simulink model "StepperMotor_time_solver_curve_caratteristiche"  (R2023b)
settings: Solver=FixedStepDiscrete  StartTime=0.0  StopTime=0.25  FixedStep=Ts  MaxStep=2e-6  EnableMultiTasking=on
PreLoadFcn:
  | assignin('base','Ts',1e-6);
InitFcn:
  | Ts=1e-6;
undefined symbols (not defined in the file or in its folder): DiscIntNeverNeededParam
libraries: spsUniversalBridgeLib x2, spsCurrentMeasurementLib x2, spsDCVoltageSourceLib x1, spsStepperMotorLib x1, SignalEditorBlockLib x1, spspowerguiLib x1
settings Model: Creator=The MathWorks, Inc.  LastModifiedBy=simon
settings SolverCC: AlgebraicLoopSolver=TrustRegion
settings DataIOCC: LimitDataPoints=on  SaveFormat=Array  ReturnWorkspaceOutputs=off
settings OptimizationCC: ExpressionDepthLimit=2147483647  InitFltsAndDblsToZero=on  LifeSpan=inf
settings DebuggingCC: UnderspecifiedInitializationDetection=Classic  MergeDetectMultiDrivingBlocksExec=none  SignalResolutionControl=TryResolveAllWithWarning  SolverPrmCheckMsg=warning  FcnCallInpInsideContextMsg=warning  UnconnectedInputMsg=warning  UnconnectedOutputMsg=warning  UnconnectedLineMsg=warning  StateNameClashWarn=warning  SubsystemReferenceDiagnosticForUnitTest=warning  SFUnexpectedBacktrackingDiag=warning  SFNoUnconditionalDefaultTransitionDiag=warning  SFExecutionAtInitializationDiag=none  ArithmeticOperatorsInVariantConditions=warning
settings HardwareCC: ProdBitPerPointer=32  ProdBitPerSizeT=32  ProdBitPerPtrDiffT=32  ProdLargestAtomicFloat=None  ProdIntDivRoundTo=Undefined  ProdEndianess=Unspecified  ProdWordSize=32  ProdHWDeviceType=32-bit Generic
settings ModelReferenceCC: EnableRefExpFcnMdlSchedulingChecks=on  PropagateSignalLabelsOutOfModel=off
settings SFSimCC: SimUseLocalCustomCode=off  CustomCodeUndefinedFunction=UseInterfaceOnly
settings RTWCC: RTWUseLocalCustomCode=off  DLArmComputeVersion=19.05
settings CodeAppCC: StateflowObjectComments=on
settings GRTTargetCC: TargetLangStandard=C89/C90 (ANSI)  CombineOutputUpdateFcns=off  GRTInterface=on
settings ConfigComp: CovMetricSettings=dw  CovSaveCumulativeToWorkspaceVar=on  CovSaveSingleToWorkspaceVar=on  CovExternalEMLEnable=off  CovSFcnEnable=off
settings SimscapeCC: SimscapeNormalizeSystem=off

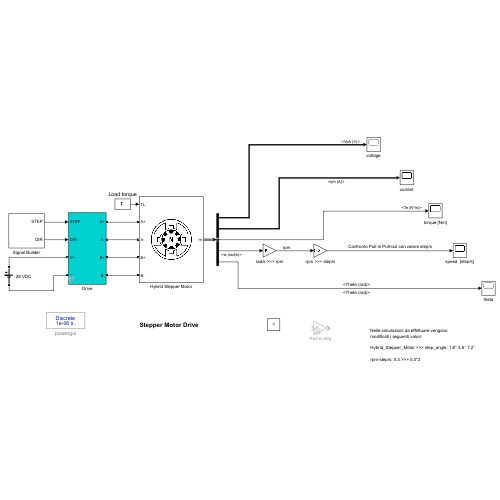
[thumbnail: Simulink's stored preview of the top-level diagram]
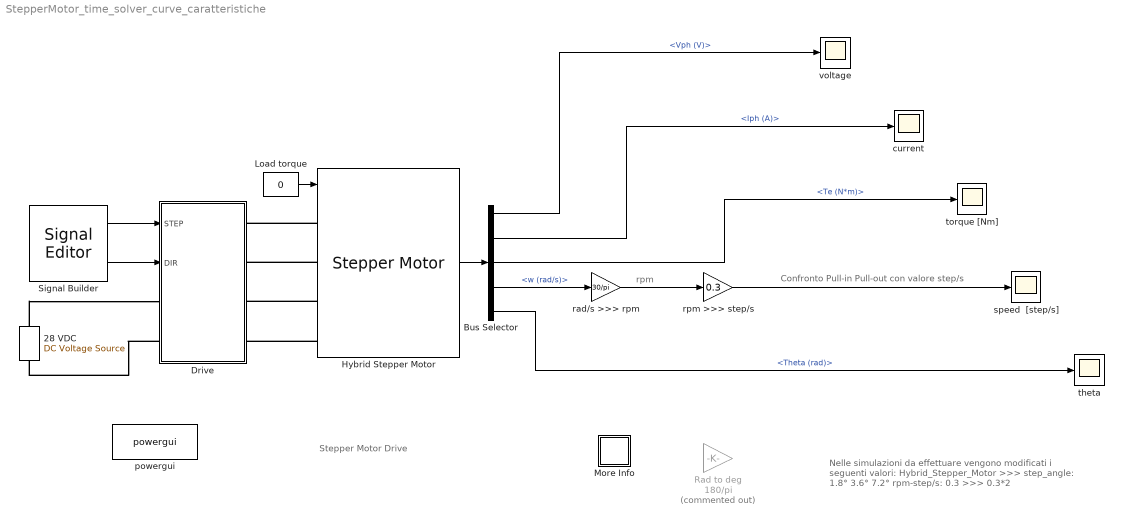
== system StepperMotor_time_solver_curve_caratteristiche ==
  note: Nelle simulazioni da effettuare vengono
      | modificati i seguenti valori:
      |
      | Hybrid_Stepper_Motor >>> step_angle: 1.8° 3.6° 7.2°
      |
      | rpm-step/s: 0.3 >>> 0.3*2
  note: Confronto Pull-in Pull-out con valore step/s
  note: rpm
  note: Stepper Motor Drive
  28 VDC : spsDCVoltageSourceLib/DC Voltage Source  Amplitude=28  Measurements=None
  Bus Selector : BusSelector  OutputSignals=Vph (V),Iph (A),Te (N*m),w (rad/s),Theta (rad)
  Drive : Subsystem  mask{Iref=2, step=500, Ts=Ts}
      mask prompts: Iref "Phase current (A)"; step "Stepping rate (step/s)"; Ts "Sampling time (s)"
      mask init:
      | Nstep=round(1/step/Ts);
  Hybrid Stepper Motor : spsStepperMotorLib/Stepper Motor  MotorType=Permanent-magnet / Hybrid  NumberOfPhases_1=2  NumberOfPhases_2=3  PresetModel_1=<empty>  PresetModel_2=<empty>  L=1.4e-3  Lmax=10e-3  Lmin=2e-3  R=0.7  Step_angle=1.8  Psim=0.005  Tdm=0.002  J=1.2e-7  B=1e-7*1000  w0=0  pos0=0  TsPowergui=0  TsBlock=-1
  Load torque : Constant  Value=0
  More Info : Subsystem
      settings: OpenFcn="showExample(\"simscapeelectricalsps/StepperMotorExample\")"
      mask Display: disp('?')
  Rad to deg : Gain  Commented=on  Gain=180/pi
  Signal Builder : SignalEditorBlockLib/Signal Editor  FileName=StepperMotorData.mat  ActiveScenario=Group_1  ActiveSignal=DIR  IsBus=off  OutputBusObjectStr=Bus: BusObject  SampleTime=0  OutputAfterFinalValue=Extrapolation  Unit=inherit  PreserveSignalName=on  ApplySigPropsToAllScenarios=on  ApplySigPropsToAllSignals=off
  current : Scope
  powergui : spspowerguiLib/powergui  SimulationMode=Discrete  SampleTime=Ts  frequency=60  Iterations=50  frequencyindice=0  Pbase=100e6  ErrMax=1e-4  UnitsV=kV  UnitsW=MW  buscounter=0  FunctionMessages=off  echomessages=off  EnableUseOfTLC=off  CurrentSourceSwitches=off  DisableSnubberDevices=off  DisableRonSwitches=off  DisableVfSwitches=off  DisplayEquations=off  AutomaticDiscreteSolvers=off  SolverType=Tustin/Backward Euler (TBE)  Interpol=off  ExternalGateDelay=off  methode=off  Ts=0  x0status=blocks  SPID=off  SwTol=0  HookPort=off  NonlinearTolerance=1e-4  nMaxIteration=100  ContinueOnMaxIteration=off  RestoreLinks=warning  ResistiveCurrentMeasurement=off  Frange=[0:2:500]  Ylog=off  Xlog=on  ShowGrid=off  save=off  variable=ZData  structure=0  ZoomFFT=on  StartTime=0.0  cycles=1  DisplayStyle=1  fundamental=60  FreqAxis=off  MaxFrequency=1000  frequencyindicesteady=1  RmsSteady=1  display=off
  rad/s >>> rpm : Gain  Gain=30/pi
  rpm >>> step/s : Gain  Gain=0.3
  speed  [step/s] : Scope
  theta : Scope
  torque [Nm] : Scope
  voltage : Scope
  wires:
  Load torque/1 -> Hybrid Stepper Motor/1
  Hybrid Stepper Motor/1 -> Bus Selector/1
  Bus Selector/1 -> voltage/1  "<Vph (V)>"
  Bus Selector/2 -> current/1  "<Iph (A)>"
  Bus Selector/3 -> torque [Nm]/1  "<Te (N*m)>"
  Bus Selector/5 -> theta/1  "<Theta (rad)>"
  Signal Builder/1 -> Drive/1(STEP)
  Signal Builder/2 -> Drive/2(DIR)
  Bus Selector/4 -> rad/s >>> rpm/1  "<w (rad/s)>"
  rad/s >>> rpm/1 -> rpm >>> step/s/1
  rpm >>> step/s/1 -> speed  [step/s]/1
  connections:
  Hybrid Stepper Motor/LConn2 -- Drive/RConn2
  Hybrid Stepper Motor/LConn3 -- Drive/RConn3
  Hybrid Stepper Motor/LConn1 -- Drive/RConn1
  Drive/LConn2 -- 28 VDC/LConn1
  28 VDC/RConn1 -- Drive/LConn1
  Hybrid Stepper Motor/LConn4 -- Drive/RConn4

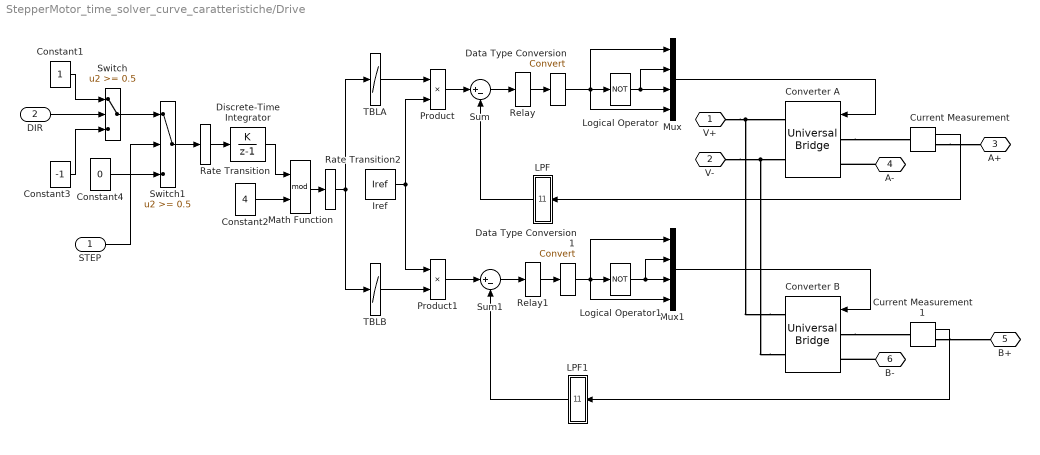
== system StepperMotor_time_solver_curve_caratteristiche/Drive ==
  STEP : Inport
  DIR : Inport  Port=2
  Constant1 : Constant  SampleTime=Ts
  Constant2 : Constant  Value=4  SampleTime=Nstep*Ts
  Constant3 : Constant  Value=-1  SampleTime=Ts
  Constant4 : Constant  Value=0  SampleTime=Ts
  Converter A : spsUniversalBridgeLib/Universal Bridge  Arms=2  SnubberResistance=10000  SnubberCapacitance=inf  Device=MOSFET / Diodes  Ron=1e-3*10  Lon=0  ForwardVoltages="[  0  0  ]"  ForwardVoltage=0  GTOparameters=[ 10e-6 , 20e-6 ]  IGBTparameters=[ 0.5e-6 , 0.5e-6 ]  Measurements=None  Measurements_2=None  converterType=Rectifier
  Converter B : spsUniversalBridgeLib/Universal Bridge  Arms=2  SnubberResistance=10000  SnubberCapacitance=inf  Device=MOSFET / Diodes  Ron=1e-3*10  Lon=0  ForwardVoltages="[  0  0  ]"  ForwardVoltage=0  GTOparameters=[ 10e-6 , 20e-6 ]  IGBTparameters=[ 0.5e-6 , 0.5e-6 ]  Measurements=None  Measurements_2=None  converterType=Rectifier
  Current Measurement : spsCurrentMeasurementLib/Current Measurement  PhasorSimulation=off  OutputType=Complex  PSBequivalent=0
  Current Measurement1 : spsCurrentMeasurementLib/Current Measurement  PhasorSimulation=off  OutputType=Complex  PSBequivalent=0
  Data Type Conversion : DataTypeConversion  SaturateOnIntegerOverflow=off  RndMeth=Floor
  Data Type Conversion1 : DataTypeConversion  SaturateOnIntegerOverflow=off  RndMeth=Floor
  Discrete-Time Integrator : DiscreteIntegrator  IntegratorMethod=Accumulation: Forward Euler  SampleTime=Nstep*Ts  ICPrevOutput=DiscIntNeverNeededParam  ICPrevScaledInput=DiscIntNeverNeededParam
  Iref : Constant  Value=Iref  SampleTime=Ts
  LPF : Subsystem  mask{fc=10000, Ts=Ts}
      mask prompts: fc "Cut-off frequency (Hz)"; Ts "Sampling time (s)"
      mask init:
      | % fa=tf(1,[1/2/pi/fc 1]);
      | % fn=c2d(fa,Ts);
      | % [NN,DD]=tfdata(fn,'v')
      | 
      | NN = [ 0,0.0609];
      | DD = [1.0000,-0.9391];
  LPF1 : Subsystem  mask{fc=10000, Ts=Ts}
      mask prompts: fc "Cut-off frequency (Hz)"; Ts "Sampling time (s)"
      mask init:
      | % fa=tf(1,[1/2/pi/fc 1]);
      | % fn=c2d(fa,Ts);
      | % [NN,DD]=tfdata(fn,'v')
      | 
      | NN = [ 0,0.0609];
      | DD = [1.0000,-0.9391];
  Logical Operator : Logic  Operator=NOT  AllPortsSameDT=off  OutDataTypeStr=boolean
  Logical Operator1 : Logic  Operator=NOT  AllPortsSameDT=off  OutDataTypeStr=boolean
  Math Function : Math  Operator=mod  SignedPower=on  SampleTime=Nstep*Ts
  Mux : Mux
  Mux1 : Mux
  Product : Product  RndMeth=Zero
  Product1 : Product  RndMeth=Zero
  Rate Transition : RateTransition
  Rate Transition2 : RateTransition
  Relay : Relay  OnSwitchValue=0.01  OffSwitchValue=-0.01
  Relay1 : Relay  OnSwitchValue=0.01  OffSwitchValue=-0.01  OutDataTypeStr=Inherit: Inherit via back propagation
  Sum : Sum  Inputs=|+-  OutDataTypeStr=Inherit: Same as first input
  Sum1 : Sum  Inputs=|+-  OutDataTypeStr=Inherit: Same as first input
  Switch : Switch  Threshold=0.5  ZeroCross=off  SampleTime=Ts  SaturateOnIntegerOverflow=off  InputSameDT=off
  Switch1 : Switch  Threshold=0.5  ZeroCross=off  SampleTime=Ts  SaturateOnIntegerOverflow=off  InputSameDT=off
  TBLA : Lookup_n-D  NumberOfTableDimensions=1  BreakpointsForDimension1=[0:3]  BreakpointsForDimension2=[0 571.55 685.8 800.15 914.4 1028.8 1143.1 1257.4 1371.7 1486 1600.3 1714.6 1828.9 1943.2 2057.5 2171.8 2286.1 2400.5 2514.7 2629.1 2743.3 2857.7 2971.9 3086.3 3200.5 3314.9 3429.2]  Table=[1 0 -1 0]  InternalRulePriority=Speed  RndMeth=Simplest
  TBLB : Lookup_n-D  NumberOfTableDimensions=1  BreakpointsForDimension1=[0:3]  BreakpointsForDimension2=[0 571.55 685.8 800.15 914.4 1028.8 1143.1 1257.4 1371.7 1486 1600.3 1714.6 1828.9 1943.2 2057.5 2171.8 2286.1 2400.5 2514.7 2629.1 2743.3 2857.7 2971.9 3086.3 3200.5 3314.9 3429.2]  Table=[0 1 0 -1]  InternalRulePriority=Speed  RndMeth=Simplest
  V+ : PMIOPort  Side=Left
  V- : PMIOPort  Port=2  Side=Left
  A+ : PMIOPort  Port=3  Side=Right
  A- : PMIOPort  Port=4  Side=Right
  B+ : PMIOPort  Port=5  Side=Right
  B- : PMIOPort  Port=6  Side=Right
  wires:
  Constant4/1 -> Switch1/3
  Switch1/1 -> Rate Transition/1
  Switch/1 -> Switch1/1
  STEP/1 -> Switch1/2
  DIR/1 -> Switch/2
  Rate Transition2/1 -> TBLB/1, TBLA/1
  Math Function/1 -> Rate Transition2/1
  Product1/1 -> Sum1/1
  Product/1 -> Sum/1
  Rate Transition/1 -> Discrete-Time Integrator/1
  Constant3/1 -> Switch/3
  Constant1/1 -> Switch/1
  Discrete-Time Integrator/1 -> Math Function/1
  Constant2/1 -> Math Function/2
  Iref/1 -> Product1/1, Product/2
  TBLB/1 -> Product1/2
  TBLA/1 -> Product/1
  LPF1/1(O) -> Sum1/2
  LPF/1(O) -> Sum/2
  Data Type Conversion1/1 -> Mux1/4, Mux1/1, Logical Operator1/1
  Data Type Conversion/1 -> Logical Operator/1, Mux/4, Mux/1
  Current Measurement1/1 -> LPF1/1(I)
  Sum1/1 -> Relay1/1
  Mux1/1 -> Converter B/1
  Logical Operator1/1 -> Mux1/2, Mux1/3
  Relay1/1 -> Data Type Conversion1/1
  Mux/1 -> Converter A/1
  Logical Operator/1 -> Mux/2, Mux/3
  Relay/1 -> Data Type Conversion/1
  Current Measurement/1 -> LPF/1(I)
  Sum/1 -> Relay/1
  connections:
  Converter B/RConn2 -- Converter A/RConn2 -- V-/RConn1
  Converter B/RConn1 -- Converter A/RConn1 -- V+/RConn1
  Current Measurement1/RConn1 -- B+/RConn1
  Converter B/LConn1 -- Current Measurement1/LConn1
  Current Measurement/RConn1 -- A+/RConn1
  Converter A/LConn1 -- Current Measurement/LConn1
  B-/RConn1 -- Converter B/LConn2
  A-/RConn1 -- Converter A/LConn2

== system StepperMotor_time_solver_curve_caratteristiche/More Info ==

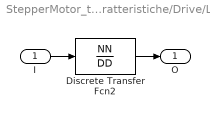
== system StepperMotor_time_solver_curve_caratteristiche/Drive/LPF ==
  I : Inport
  Discrete Transfer Fcn2 : DiscreteTransferFcn  Numerator=NN  Denominator=DD  SampleTime=Ts
  O : Outport  VectorParamsAs1DForOutWhenUnconnected=off
  wires:
  Discrete Transfer Fcn2/1 -> O/1
  I/1 -> Discrete Transfer Fcn2/1

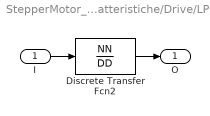
== system StepperMotor_time_solver_curve_caratteristiche/Drive/LPF1 ==
  I : Inport
  Discrete Transfer Fcn2 : DiscreteTransferFcn  Numerator=NN  Denominator=DD  SampleTime=Ts
  O : Outport  VectorParamsAs1DForOutWhenUnconnected=off
  wires:
  I/1 -> Discrete Transfer Fcn2/1
  Discrete Transfer Fcn2/1 -> O/1
